simulink model "MSBR_Plant"  (R2021b)
settings: Solver=ode45  StartTime=0.0  StopTime=sim_time  MaxStep=ts_max  RelTol=1e-4
values from neighbouring files (symbols this model uses):
  a_1 = 8.7292e-2/wilson_ratio    (= 0.0087292)    [Whole_Plant_Cool_Pump_Accident_script.m]    (also in Whole_Plant_Fert_Pump_Accident_script.m; Whole_Plant_Fuel_Pump_Accident.m; Whole_Plant_Fuel_Pump_Accident_script.m; Whole_Plant_Reactivity_Accident.m)
  a_2 = 7.3787e-4/wilson_ratio    (= 7.3787e-05)    [Whole_Plant_Cool_Pump_Accident_script.m]    (also in Whole_Plant_Fert_Pump_Accident_script.m; Whole_Plant_Fuel_Pump_Accident.m; Whole_Plant_Fuel_Pump_Accident_script.m; Whole_Plant_Reactivity_Accident.m)
  a_b = 1.656e-5    (= 1.656e-05)    [Whole_Plant_Cool_Pump_Accident_script.m]    (also in Whole_Plant_Fert_Pump_Accident_script.m; Whole_Plant_Fuel_Pump_Accident.m; Whole_Plant_Fuel_Pump_Accident_script.m; Whole_Plant_Reactivity_Accident.m)
  a_f = -8.172e-5    (= -8.172e-05)    [Whole_Plant_Cool_Pump_Accident_script.m]    (also in Whole_Plant_Fert_Pump_Accident_script.m; Whole_Plant_Fuel_Pump_Accident.m; Whole_Plant_Fuel_Pump_Accident_script.m; Whole_Plant_Reactivity_Accident.m)
  a_g = 2.016e-5    (= 2.016e-05)    [Whole_Plant_Cool_Pump_Accident_script.m]    (also in Whole_Plant_Fert_Pump_Accident_script.m; Whole_Plant_Fuel_Pump_Accident.m; Whole_Plant_Fuel_Pump_Accident_script.m; Whole_Plant_Reactivity_Accident.m)
  A_s = pi()*((D_OTSG_i^2)/4) - A_w_OTSG - A_p_OTSG    [Whole_Plant_Cool_Pump_Accident_script.m]    (also in Whole_Plant_Fert_Pump_Accident_script.m; Whole_Plant_Fuel_Pump_Accident.m; Whole_Plant_Fuel_Pump_Accident_script.m; Whole_Plant_Reactivity_Accident.m)
  alpha_co = 316.2    [Whole_Plant_Cool_Pump_Accident_script.m]    (also in Whole_Plant_Fert_Pump_Accident_script.m; Whole_Plant_Fuel_Pump_Accident.m; Whole_Plant_Fuel_Pump_Accident_script.m; Whole_Plant_Reactivity_Accident.m)
  beta = [2.290e-04, 8.320e-04, 7.100e-04, 8.520e-04, 1.710e-04, 1.020e-04]    [Whole_Plant_Cool_Pump_Accident_script.m]    (also in Whole_Plant_Fert_Pump_Accident_script.m; Whole_Plant_Fuel_Pump_Accident.m; Whole_Plant_Fuel_Pump_Accident_script.m; Whole_Plant_Reactivity_Accident.m)
  beta_co = 68.0958    [Whole_Plant_Cool_Pump_Accident_script.m]    (also in Whole_Plant_Fert_Pump_Accident_script.m; Whole_Plant_Fuel_Pump_Accident.m; Whole_Plant_Fuel_Pump_Accident_script.m; Whole_Plant_Reactivity_Accident.m)
  beta_t = sum(beta)    [Whole_Plant_Cool_Pump_Accident_script.m]    (also in Whole_Plant_Fert_Pump_Accident_script.m; Whole_Plant_Fuel_Pump_Accident.m; Whole_Plant_Fuel_Pump_Accident_script.m; Whole_Plant_Reactivity_Accident.m)
  C_nc_X_A_nc = 12.8    [Whole_Plant_Cool_Pump_Accident_script.m]    (also in Whole_Plant_Fert_Pump_Accident_script.m; Whole_Plant_Fuel_Pump_Accident.m; Whole_Plant_Fuel_Pump_Accident_script.m; Whole_Plant_Reactivity_Accident.m)
  C_pcw = 0.0042    [Whole_Plant_Cool_Pump_Accident_script.m]    (also in Whole_Plant_Fert_Pump_Accident_script.m; Whole_Plant_Fuel_Pump_Accident.m; Whole_Plant_Fuel_Pump_Accident_script.m; Whole_Plant_Reactivity_Accident.m)
  C_rh_X_A_rh = 33    [Whole_Plant_Cool_Pump_Accident_script.m]    (also in Whole_Plant_Fert_Pump_Accident_script.m; Whole_Plant_Fuel_Pump_Accident.m; Whole_Plant_Fuel_Pump_Accident_script.m; Whole_Plant_Reactivity_Accident.m)
  C_v = 0.84    [Whole_Plant_Cool_Pump_Accident_script.m]    (also in Whole_Plant_Fert_Pump_Accident_script.m; Whole_Plant_Fuel_Pump_Accident.m; Whole_Plant_Fuel_Pump_Accident_script.m; Whole_Plant_Reactivity_Accident.m)
  ce1 = 1.2471e-07    [Whole_Plant_Cool_Pump_Accident_script.m]    (also in Whole_Plant_Fert_Pump_Accident_script.m; Whole_Plant_Fuel_Pump_Accident.m; Whole_Plant_Fuel_Pump_Accident_script.m; Whole_Plant_Reactivity_Accident.m)
  ce2 = 5.3816e-14    [Whole_Plant_Cool_Pump_Accident_script.m]    (also in Whole_Plant_Fert_Pump_Accident_script.m; Whole_Plant_Fuel_Pump_Accident.m; Whole_Plant_Fuel_Pump_Accident_script.m; Whole_Plant_Reactivity_Accident.m)
  ce3 = 3.3721e-08    [Whole_Plant_Cool_Pump_Accident_script.m]    (also in Whole_Plant_Fert_Pump_Accident_script.m; Whole_Plant_Fuel_Pump_Accident.m; Whole_Plant_Fuel_Pump_Accident_script.m; Whole_Plant_Reactivity_Accident.m)
  Cp_fw = XSteam('Cp_pT',P_set*10,T_fw)/1000    [Whole_Plant_Cool_Pump_Accident_script.m]    (also in Whole_Plant_Fert_Pump_Accident_script.m; Whole_Plant_Fuel_Pump_Accident.m; Whole_Plant_Fuel_Pump_Accident_script.m; Whole_Plant_Reactivity_Accident.m)
  Cp_p = Cp_sec    (= 0.001716588)    [Whole_Plant_Cool_Pump_Accident_script.m]    (also in Whole_Plant_Fert_Pump_Accident_script.m; Whole_Plant_Fuel_Pump_Accident.m; Whole_Plant_Fuel_Pump_Accident_script.m; Whole_Plant_Reactivity_Accident.m)
  Cp_rh = 0.0021520    (= 0.002152)    [Whole_Plant_Cool_Pump_Accident_script.m]    (also in Whole_Plant_Fert_Pump_Accident_script.m; Whole_Plant_Fuel_Pump_Accident.m; Whole_Plant_Fuel_Pump_Accident_script.m; Whole_Plant_Reactivity_Accident.m)
  Cp_s = XSteam('Cp_pT',P_s*10,T_s)/1000    [Whole_Plant_Cool_Pump_Accident_script.m]    (also in Whole_Plant_Fert_Pump_Accident_script.m; Whole_Plant_Fuel_Pump_Accident.m; Whole_Plant_Fuel_Pump_Accident_script.m; Whole_Plant_Reactivity_Accident.m)
  Cp_sc = XSteam('Cp_pT',P_set*10,T_sc2)/1000    [Whole_Plant_Cool_Pump_Accident_script.m]    (also in Whole_Plant_Fert_Pump_Accident_script.m; Whole_Plant_Fuel_Pump_Accident.m; Whole_Plant_Fuel_Pump_Accident_script.m; Whole_Plant_Reactivity_Accident.m)
  Cp_w = 468.992e-6    (= 0.000468992)    [Whole_Plant_Cool_Pump_Accident_script.m]    (also in Whole_Plant_Fert_Pump_Accident_script.m; Whole_Plant_Fuel_Pump_Accident.m; Whole_Plant_Fuel_Pump_Accident_script.m; Whole_Plant_Reactivity_Accident.m)
  D_it = D_ot-2*T_th    (= 0.014147)    [Whole_Plant_Cool_Pump_Accident_script.m]    (also in Whole_Plant_Fert_Pump_Accident_script.m; Whole_Plant_Fuel_Pump_Accident.m; Whole_Plant_Fuel_Pump_Accident_script.m; Whole_Plant_Reactivity_Accident.m)
  D_ot = 0.015875    [Whole_Plant_Cool_Pump_Accident_script.m]    (also in Whole_Plant_Fert_Pump_Accident_script.m; Whole_Plant_Fuel_Pump_Accident.m; Whole_Plant_Fuel_Pump_Accident_script.m; Whole_Plant_Reactivity_Accident.m)
  dHs_dPs = c(1)    [Whole_Plant_Cool_Pump_Accident_script.m]    (also in Whole_Plant_Fert_Pump_Accident_script.m; Whole_Plant_Fuel_Pump_Accident.m; Whole_Plant_Fuel_Pump_Accident_script.m; Whole_Plant_Reactivity_Accident.m)
  eta_hp_isen = 0.861    [Whole_Plant_Cool_Pump_Accident_script.m]    (also in Whole_Plant_Fert_Pump_Accident_script.m; Whole_Plant_Fuel_Pump_Accident.m; Whole_Plant_Fuel_Pump_Accident_script.m; Whole_Plant_Reactivity_Accident.m)
  eta_lp_isen = 0.861    [Whole_Plant_Cool_Pump_Accident_script.m]    (also in Whole_Plant_Fert_Pump_Accident_script.m; Whole_Plant_Fuel_Pump_Accident.m; Whole_Plant_Fuel_Pump_Accident_script.m; Whole_Plant_Reactivity_Accident.m)
  gamma_I = 5.1135e-2    (= 0.051135)    [Whole_Plant_Cool_Pump_Accident_script.m]    (also in Whole_Plant_Fert_Pump_Accident_script.m; Whole_Plant_Fuel_Pump_Accident.m; Whole_Plant_Fuel_Pump_Accident_script.m; Whole_Plant_Reactivity_Accident.m)
  gamma_Xe = 1.1628e-2    (= 0.011628)    [Whole_Plant_Cool_Pump_Accident_script.m]    (also in Whole_Plant_Fert_Pump_Accident_script.m; Whole_Plant_Fuel_Pump_Accident.m; Whole_Plant_Fuel_Pump_Accident_script.m; Whole_Plant_Reactivity_Accident.m)
  H_co0 = 0.149    [Whole_Plant_Cool_Pump_Accident_script.m]    (also in Whole_Plant_Fert_Pump_Accident_script.m; Whole_Plant_Fuel_Pump_Accident.m; Whole_Plant_Fuel_Pump_Accident_script.m; Whole_Plant_Reactivity_Accident.m)
  H_f_co0 = 0.149    [Whole_Plant_Cool_Pump_Accident_script.m]    (also in Whole_Plant_Fert_Pump_Accident_script.m; Whole_Plant_Fuel_Pump_Accident.m; Whole_Plant_Fuel_Pump_Accident_script.m; Whole_Plant_Reactivity_Accident.m)
  H_fg_co0 = 2.35    [Whole_Plant_Cool_Pump_Accident_script.m]    (also in Whole_Plant_Fert_Pump_Accident_script.m; Whole_Plant_Fuel_Pump_Accident.m; Whole_Plant_Fuel_Pump_Accident_script.m; Whole_Plant_Reactivity_Accident.m)
  H_fgrh0 = (XSteam('hV_p', P_s*1e1) - XSteam('hL_p', P_s*1e1))/1e3    [Whole_Plant_Cool_Pump_Accident_script.m]    (also in Whole_Plant_Fert_Pump_Accident_script.m; Whole_Plant_Fuel_Pump_Accident.m; Whole_Plant_Fuel_Pump_Accident_script.m; Whole_Plant_Reactivity_Accident.m)
  H_frh0 = XSteam('hL_p', P_s*1e1)/1e3    [Whole_Plant_Cool_Pump_Accident_script.m]    (also in Whole_Plant_Fert_Pump_Accident_script.m; Whole_Plant_Fuel_Pump_Accident.m; Whole_Plant_Fuel_Pump_Accident_script.m; Whole_Plant_Reactivity_Accident.m)
  h_fwh1 = 0.5927    [Whole_Plant_Cool_Pump_Accident_script.m]    (also in Whole_Plant_Fert_Pump_Accident_script.m; Whole_Plant_Fuel_Pump_Accident.m; Whole_Plant_Fuel_Pump_Accident_script.m; Whole_Plant_Reactivity_Accident.m)
  H_fwh10 = 0.46009    [Whole_Plant_Cool_Pump_Accident_script.m]    (also in Whole_Plant_Fert_Pump_Accident_script.m; Whole_Plant_Fuel_Pump_Accident.m; Whole_Plant_Fuel_Pump_Accident_script.m; Whole_Plant_Reactivity_Accident.m)
  h_fwh2 = 1.230803    [Whole_Plant_Cool_Pump_Accident_script.m]    (also in Whole_Plant_Fert_Pump_Accident_script.m; Whole_Plant_Fuel_Pump_Accident.m; Whole_Plant_Fuel_Pump_Accident_script.m; Whole_Plant_Reactivity_Accident.m)
  H_fwh20 = 0.6784    [Whole_Plant_Cool_Pump_Accident_script.m]    (also in Whole_Plant_Fert_Pump_Accident_script.m; Whole_Plant_Fuel_Pump_Accident.m; Whole_Plant_Fuel_Pump_Accident_script.m; Whole_Plant_Reactivity_Accident.m)
  H_grh0 = 2.8029    [Whole_Plant_Cool_Pump_Accident_script.m]    (also in Whole_Plant_Fert_Pump_Accident_script.m; Whole_Plant_Fuel_Pump_Accident.m; Whole_Plant_Fuel_Pump_Accident_script.m; Whole_Plant_Reactivity_Accident.m)
  H_hp_isen0 = 2.5111    [Whole_Plant_Cool_Pump_Accident_script.m]    (also in Whole_Plant_Fert_Pump_Accident_script.m; Whole_Plant_Fuel_Pump_Accident.m; Whole_Plant_Fuel_Pump_Accident_script.m; Whole_Plant_Reactivity_Accident.m)
  H_hpt_out = 2.6201    [Whole_Plant_Cool_Pump_Accident_script.m]    (also in Whole_Plant_Fert_Pump_Accident_script.m; Whole_Plant_Fuel_Pump_Accident.m; Whole_Plant_Fuel_Pump_Accident_script.m; Whole_Plant_Reactivity_Accident.m)
  H_lp_isen = 958.4*1054.35e-6/0.45359237    (= 2.22774699671)    [Whole_Plant_Cool_Pump_Accident_script.m]    (also in Whole_Plant_Fert_Pump_Accident_script.m; Whole_Plant_Fuel_Pump_Accident.m; Whole_Plant_Fuel_Pump_Accident_script.m; Whole_Plant_Reactivity_Accident.m)
  H_lpt_out = 2.3089    [Whole_Plant_Cool_Pump_Accident_script.m]    (also in Whole_Plant_Fert_Pump_Accident_script.m; Whole_Plant_Fuel_Pump_Accident.m; Whole_Plant_Fuel_Pump_Accident_script.m; Whole_Plant_Reactivity_Accident.m)
  H_nc = XSteam('h_pT', P_s*10, T_s)/1000    [Whole_Plant_Cool_Pump_Accident_script.m]    (also in Whole_Plant_Fert_Pump_Accident_script.m; Whole_Plant_Fuel_Pump_Accident.m; Whole_Plant_Fuel_Pump_Accident_script.m; Whole_Plant_Reactivity_Accident.m)
  h_pw = h_s    (= 0.02555)    [Whole_Plant_Cool_Pump_Accident_script.m]    (also in Whole_Plant_Fert_Pump_Accident_script.m; Whole_Plant_Fuel_Pump_Accident.m; Whole_Plant_Fuel_Pump_Accident_script.m; Whole_Plant_Reactivity_Accident.m)
  H_rh = 2.8115    [Whole_Plant_Cool_Pump_Accident_script.m]    (also in Whole_Plant_Fert_Pump_Accident_script.m; Whole_Plant_Fuel_Pump_Accident.m; Whole_Plant_Fuel_Pump_Accident_script.m; Whole_Plant_Reactivity_Accident.m)
  h_wb = 13349.334646671E-6    (= 0.0133493346467)    [Whole_Plant_Cool_Pump_Accident_script.m]    (also in Whole_Plant_Fert_Pump_Accident_script.m; Whole_Plant_Fuel_Pump_Accident.m; Whole_Plant_Fuel_Pump_Accident_script.m; Whole_Plant_Reactivity_Accident.m)
  h_ws = 5732.378387768E-6    (= 0.00573237838777)    [Whole_Plant_Cool_Pump_Accident_script.m]    (also in Whole_Plant_Fert_Pump_Accident_script.m; Whole_Plant_Fuel_Pump_Accident.m; Whole_Plant_Fuel_Pump_Accident_script.m; Whole_Plant_Reactivity_Accident.m)
  h_wsc = 8385.005556375E-6    (= 0.00838500555638)    [Whole_Plant_Cool_Pump_Accident_script.m]    (also in Whole_Plant_Fert_Pump_Accident_script.m; Whole_Plant_Fuel_Pump_Accident.m; Whole_Plant_Fuel_Pump_Accident_script.m; Whole_Plant_Reactivity_Accident.m)
  hA_bg = A_fert*h_bg    (= 2.76411813627)    [Whole_Plant_Cool_Pump_Accident_script.m]    (also in Whole_Plant_Fert_Pump_Accident_script.m; Whole_Plant_Fuel_Pump_Accident.m; Whole_Plant_Fuel_Pump_Accident_script.m; Whole_Plant_Reactivity_Accident.m)
  hA_co0 = 140    [Whole_Plant_Cool_Pump_Accident_script.m]    (also in Whole_Plant_Fert_Pump_Accident_script.m; Whole_Plant_Fuel_Pump_Accident.m; Whole_Plant_Fuel_Pump_Accident_script.m; Whole_Plant_Reactivity_Accident.m)
  hA_fg_dn = h_fg*A_fuel_down    [Whole_Plant_Cool_Pump_Accident_script.m]    (also in Whole_Plant_Fert_Pump_Accident_script.m; Whole_Plant_Fuel_Pump_Accident.m; Whole_Plant_Fuel_Pump_Accident_script.m; Whole_Plant_Reactivity_Accident.m)
  hA_fg_up = h_fg*A_fuel_up    [Whole_Plant_Cool_Pump_Accident_script.m]    (also in Whole_Plant_Fert_Pump_Accident_script.m; Whole_Plant_Fuel_Pump_Accident.m; Whole_Plant_Fuel_Pump_Accident_script.m; Whole_Plant_Reactivity_Accident.m)
  hA_p_bhx1 = [h_pb*A_pbhx/2,h_pb*A_pbhx/2]    [Whole_Plant_Cool_Pump_Accident_script.m]    (also in Whole_Plant_Fert_Pump_Accident_script.m; Whole_Plant_Fuel_Pump_Accident.m; Whole_Plant_Fuel_Pump_Accident_script.m; Whole_Plant_Reactivity_Accident.m)
  hA_p_bhx2 = hA_p_bhx1    [Whole_Plant_Cool_Pump_Accident_script.m]    (also in Whole_Plant_Fert_Pump_Accident_script.m; Whole_Plant_Fuel_Pump_Accident.m; Whole_Plant_Fuel_Pump_Accident_script.m; Whole_Plant_Reactivity_Accident.m)
  hA_p_bhx3 = hA_p_bhx1    [Whole_Plant_Cool_Pump_Accident_script.m]    (also in Whole_Plant_Fert_Pump_Accident_script.m; Whole_Plant_Fuel_Pump_Accident.m; Whole_Plant_Fuel_Pump_Accident_script.m; Whole_Plant_Reactivity_Accident.m)
  hA_p_bhx4 = hA_p_bhx1    [Whole_Plant_Cool_Pump_Accident_script.m]    (also in Whole_Plant_Fert_Pump_Accident_script.m; Whole_Plant_Fuel_Pump_Accident.m; Whole_Plant_Fuel_Pump_Accident_script.m; Whole_Plant_Reactivity_Accident.m)
  hA_p_fhx1 = [h_p*A_pfhx_dn/2,h_p*A_pfhx_dn/2,h_p*A_pfhx_up/2,h_p*A_pfhx_up/2]    [Whole_Plant_Cool_Pump_Accident_script.m]    (also in Whole_Plant_Fert_Pump_Accident_script.m; Whole_Plant_Fuel_Pump_Accident.m; Whole_Plant_Fuel_Pump_Accident_script.m; Whole_Plant_Reactivity_Accident.m)
  hA_p_fhx2 = hA_p_fhx1    [Whole_Plant_Cool_Pump_Accident_script.m]    (also in Whole_Plant_Fert_Pump_Accident_script.m; Whole_Plant_Fuel_Pump_Accident.m; Whole_Plant_Fuel_Pump_Accident_script.m; Whole_Plant_Reactivity_Accident.m)
  hA_p_fhx3 = hA_p_fhx1    [Whole_Plant_Cool_Pump_Accident_script.m]    (also in Whole_Plant_Fert_Pump_Accident_script.m; Whole_Plant_Fuel_Pump_Accident.m; Whole_Plant_Fuel_Pump_Accident_script.m; Whole_Plant_Reactivity_Accident.m)
  hA_p_fhx4 = hA_p_fhx1    [Whole_Plant_Cool_Pump_Accident_script.m]    (also in Whole_Plant_Fert_Pump_Accident_script.m; Whole_Plant_Fuel_Pump_Accident.m; Whole_Plant_Fuel_Pump_Accident_script.m; Whole_Plant_Reactivity_Accident.m)
  hA_s_bhx1 = [h_sb*A_sbhx/2,h_sb*A_sbhx/2]    [Whole_Plant_Cool_Pump_Accident_script.m]    (also in Whole_Plant_Fert_Pump_Accident_script.m; Whole_Plant_Fuel_Pump_Accident.m; Whole_Plant_Fuel_Pump_Accident_script.m; Whole_Plant_Reactivity_Accident.m)
  hA_s_bhx2 = hA_s_bhx1    [Whole_Plant_Cool_Pump_Accident_script.m]    (also in Whole_Plant_Fert_Pump_Accident_script.m; Whole_Plant_Fuel_Pump_Accident.m; Whole_Plant_Fuel_Pump_Accident_script.m; Whole_Plant_Reactivity_Accident.m)
  hA_s_bhx3 = hA_s_bhx1    [Whole_Plant_Cool_Pump_Accident_script.m]    (also in Whole_Plant_Fert_Pump_Accident_script.m; Whole_Plant_Fuel_Pump_Accident.m; Whole_Plant_Fuel_Pump_Accident_script.m; Whole_Plant_Reactivity_Accident.m)
  hA_s_bhx4 = hA_s_bhx1    [Whole_Plant_Cool_Pump_Accident_script.m]    (also in Whole_Plant_Fert_Pump_Accident_script.m; Whole_Plant_Fuel_Pump_Accident.m; Whole_Plant_Fuel_Pump_Accident_script.m; Whole_Plant_Reactivity_Accident.m)
  hA_s_fhx1 = [h_s*A_sfhx_up/2,h_s*A_sfhx_up/2,h_s*A_sfhx_dn/2,h_s*A_sfhx_dn/2]    [Whole_Plant_Cool_Pump_Accident_script.m]    (also in Whole_Plant_Fert_Pump_Accident_script.m; Whole_Plant_Fuel_Pump_Accident.m; Whole_Plant_Fuel_Pump_Accident_script.m; Whole_Plant_Reactivity_Accident.m)
  hA_s_fhx2 = hA_s_fhx1    [Whole_Plant_Cool_Pump_Accident_script.m]    (also in Whole_Plant_Fert_Pump_Accident_script.m; Whole_Plant_Fuel_Pump_Accident.m; Whole_Plant_Fuel_Pump_Accident_script.m; Whole_Plant_Reactivity_Accident.m)
  hA_s_fhx3 = hA_s_fhx1    [Whole_Plant_Cool_Pump_Accident_script.m]    (also in Whole_Plant_Fert_Pump_Accident_script.m; Whole_Plant_Fuel_Pump_Accident.m; Whole_Plant_Fuel_Pump_Accident_script.m; Whole_Plant_Reactivity_Accident.m)
  hA_s_fhx4 = hA_s_fhx1    [Whole_Plant_Cool_Pump_Accident_script.m]    (also in Whole_Plant_Fert_Pump_Accident_script.m; Whole_Plant_Fuel_Pump_Accident.m; Whole_Plant_Fuel_Pump_Accident_script.m; Whole_Plant_Reactivity_Accident.m)
  I_0 = gamma_I*Sigma_f_msbr*phi_0/lam_I    (= 1.30000734126e+17)    [Whole_Plant_Cool_Pump_Accident_script.m]    (also in Whole_Plant_Fert_Pump_Accident_script.m; Whole_Plant_Fuel_Pump_Accident.m; Whole_Plant_Fuel_Pump_Accident_script.m; Whole_Plant_Reactivity_Accident.m)
  k_1 = 0.5    [Whole_Plant_Cool_Pump_Accident_script.m]    (also in Whole_Plant_Fert_Pump_Accident_script.m; Whole_Plant_Fuel_Pump_Accident.m; Whole_Plant_Fuel_Pump_Accident_script.m; Whole_Plant_Reactivity_Accident.m)
  K_1 = e(1)    [Whole_Plant_Cool_Pump_Accident_script.m]    (also in Whole_Plant_Fert_Pump_Accident_script.m; Whole_Plant_Fuel_Pump_Accident.m; Whole_Plant_Fuel_Pump_Accident_script.m; Whole_Plant_Reactivity_Accident.m)
  k_1b = 0.5    [Whole_Plant_Cool_Pump_Accident_script.m]    (also in Whole_Plant_Fert_Pump_Accident_script.m; Whole_Plant_Fuel_Pump_Accident.m; Whole_Plant_Fuel_Pump_Accident_script.m; Whole_Plant_Reactivity_Accident.m)
  k_2 = 0.5    [Whole_Plant_Cool_Pump_Accident_script.m]    (also in Whole_Plant_Fert_Pump_Accident_script.m; Whole_Plant_Fuel_Pump_Accident.m; Whole_Plant_Fuel_Pump_Accident_script.m; Whole_Plant_Reactivity_Accident.m)
  k_2b = 0.5    [Whole_Plant_Cool_Pump_Accident_script.m]    (also in Whole_Plant_Fert_Pump_Accident_script.m; Whole_Plant_Fuel_Pump_Accident.m; Whole_Plant_Fuel_Pump_Accident_script.m; Whole_Plant_Reactivity_Accident.m)
  k_3 = 0.5    [Whole_Plant_Cool_Pump_Accident_script.m]    (also in Whole_Plant_Fert_Pump_Accident_script.m; Whole_Plant_Fuel_Pump_Accident.m; Whole_Plant_Fuel_Pump_Accident_script.m; Whole_Plant_Reactivity_Accident.m)
  k_4 = 0.5    [Whole_Plant_Cool_Pump_Accident_script.m]    (also in Whole_Plant_Fert_Pump_Accident_script.m; Whole_Plant_Fuel_Pump_Accident.m; Whole_Plant_Fuel_Pump_Accident_script.m; Whole_Plant_Reactivity_Accident.m)
  K_4 = b(1)    [Whole_Plant_Cool_Pump_Accident_script.m]    (also in Whole_Plant_Fert_Pump_Accident_script.m; Whole_Plant_Fuel_Pump_Accident.m; Whole_Plant_Fuel_Pump_Accident_script.m; Whole_Plant_Reactivity_Accident.m)
  K_5 = a(1)    [Whole_Plant_Cool_Pump_Accident_script.m]    (also in Whole_Plant_Fert_Pump_Accident_script.m; Whole_Plant_Fuel_Pump_Accident.m; Whole_Plant_Fuel_Pump_Accident_script.m; Whole_Plant_Reactivity_Accident.m)
  K_b = d(1)    [Whole_Plant_Cool_Pump_Accident_script.m]    (also in Whole_Plant_Fert_Pump_Accident_script.m; Whole_Plant_Fuel_Pump_Accident.m; Whole_Plant_Fuel_Pump_Accident_script.m; Whole_Plant_Reactivity_Accident.m)
  k_b1 = (K_B/2)/K    (= 0.0089463103122)    [Whole_Plant_Cool_Pump_Accident_script.m]    (also in Whole_Plant_Fert_Pump_Accident_script.m; Whole_Plant_Fuel_Pump_Accident.m; Whole_Plant_Fuel_Pump_Accident_script.m; Whole_Plant_Reactivity_Accident.m)
  k_b2 = k_b1    (= 0.0089463103122)    [Whole_Plant_Cool_Pump_Accident_script.m]    (also in Whole_Plant_Fert_Pump_Accident_script.m; Whole_Plant_Fuel_Pump_Accident.m; Whole_Plant_Fuel_Pump_Accident_script.m; Whole_Plant_Reactivity_Accident.m)
  K_bhp = 0.1634    [Whole_Plant_Cool_Pump_Accident_script.m]    (also in Whole_Plant_Fert_Pump_Accident_script.m; Whole_Plant_Fuel_Pump_Accident.m; Whole_Plant_Fuel_Pump_Accident_script.m; Whole_Plant_Reactivity_Accident.m)
  K_blp = 0.2174    [Whole_Plant_Cool_Pump_Accident_script.m]    (also in Whole_Plant_Fert_Pump_Accident_script.m; Whole_Plant_Fuel_Pump_Accident.m; Whole_Plant_Fuel_Pump_Accident_script.m; Whole_Plant_Reactivity_Accident.m)
  k_f1 = ((1 - K_G - K_B - K_Ba)/4)/K    (= 0.226055463576)    [Whole_Plant_Cool_Pump_Accident_script.m]    (also in Whole_Plant_Fert_Pump_Accident_script.m; Whole_Plant_Fuel_Pump_Accident.m; Whole_Plant_Fuel_Pump_Accident_script.m; Whole_Plant_Reactivity_Accident.m)
  k_f2 = k_f1    (= 0.226055463576)    [Whole_Plant_Cool_Pump_Accident_script.m]    (also in Whole_Plant_Fert_Pump_Accident_script.m; Whole_Plant_Fuel_Pump_Accident.m; Whole_Plant_Fuel_Pump_Accident_script.m; Whole_Plant_Reactivity_Accident.m)
  k_f3 = k_f1    (= 0.226055463576)    [Whole_Plant_Cool_Pump_Accident_script.m]    (also in Whole_Plant_Fert_Pump_Accident_script.m; Whole_Plant_Fuel_Pump_Accident.m; Whole_Plant_Fuel_Pump_Accident_script.m; Whole_Plant_Reactivity_Accident.m)
  k_f4 = k_f1    (= 0.226055463576)    [Whole_Plant_Cool_Pump_Accident_script.m]    (also in Whole_Plant_Fert_Pump_Accident_script.m; Whole_Plant_Fuel_Pump_Accident.m; Whole_Plant_Fuel_Pump_Accident_script.m; Whole_Plant_Reactivity_Accident.m)
  k_g1 = ((K_G*K_fuel)/2)/K    (= 0.0346590586566)    [Whole_Plant_Cool_Pump_Accident_script.m]    (also in Whole_Plant_Fert_Pump_Accident_script.m; Whole_Plant_Fuel_Pump_Accident.m; Whole_Plant_Fuel_Pump_Accident_script.m; Whole_Plant_Reactivity_Accident.m)
  k_g2 = k_g1    (= 0.0346590586566)    [Whole_Plant_Cool_Pump_Accident_script.m]    (also in Whole_Plant_Fert_Pump_Accident_script.m; Whole_Plant_Fuel_Pump_Accident.m; Whole_Plant_Fuel_Pump_Accident_script.m; Whole_Plant_Reactivity_Accident.m)
  k_g3 = (K_G*(1-K_fuel))/K    (= 0.00856740775781)    [Whole_Plant_Cool_Pump_Accident_script.m]    (also in Whole_Plant_Fert_Pump_Accident_script.m; Whole_Plant_Fuel_Pump_Accident.m; Whole_Plant_Fuel_Pump_Accident_script.m; Whole_Plant_Reactivity_Accident.m)
  K_sc = f(1)    [Whole_Plant_Cool_Pump_Accident_script.m]    (also in Whole_Plant_Fert_Pump_Accident_script.m; Whole_Plant_Fuel_Pump_Accident.m; Whole_Plant_Fuel_Pump_Accident_script.m; Whole_Plant_Reactivity_Accident.m)
  L = 22.0    (= 22)    [Whole_Plant_Cool_Pump_Accident_script.m]    (also in Whole_Plant_Fert_Pump_Accident_script.m; Whole_Plant_Fuel_Pump_Accident.m; Whole_Plant_Fuel_Pump_Accident_script.m; Whole_Plant_Reactivity_Accident.m)
  L_b = 1.9    [Whole_Plant_Cool_Pump_Accident_script.m]    (also in Whole_Plant_Fert_Pump_Accident_script.m; Whole_Plant_Fuel_Pump_Accident.m; Whole_Plant_Fuel_Pump_Accident_script.m; Whole_Plant_Reactivity_Accident.m)
  L_s = 16.53    [Whole_Plant_Cool_Pump_Accident_script.m]    (also in Whole_Plant_Fert_Pump_Accident_script.m; Whole_Plant_Fuel_Pump_Accident.m; Whole_Plant_Fuel_Pump_Accident_script.m; Whole_Plant_Reactivity_Accident.m)
  L_sc = L-L_b-L_s    (= 3.57)    [Whole_Plant_Cool_Pump_Accident_script.m]    (also in Whole_Plant_Fert_Pump_Accident_script.m; Whole_Plant_Fuel_Pump_Accident.m; Whole_Plant_Fuel_Pump_Accident_script.m; Whole_Plant_Reactivity_Accident.m)
  Lam = 3.3e-4    (= 0.00033)    [Whole_Plant_Cool_Pump_Accident_script.m]    (also in Whole_Plant_Fert_Pump_Accident_script.m; Whole_Plant_Fuel_Pump_Accident.m; Whole_Plant_Fuel_Pump_Accident_script.m; Whole_Plant_Reactivity_Accident.m)
  lam = [1.260e-02, 3.370e-02, 1.390e-01, 3.250e-01, 1.130e+00, 2.500e+00]    [Whole_Plant_Cool_Pump_Accident_script.m]    (also in Whole_Plant_Fert_Pump_Accident_script.m; Whole_Plant_Fuel_Pump_Accident.m; Whole_Plant_Fuel_Pump_Accident_script.m; Whole_Plant_Reactivity_Accident.m)
  lam_bubl = 2.0e-2    (= 0.02)    [Whole_Plant_Cool_Pump_Accident_script.m]    (also in Whole_Plant_Fert_Pump_Accident_script.m; Whole_Plant_Fuel_Pump_Accident.m; Whole_Plant_Fuel_Pump_Accident_script.m; Whole_Plant_Reactivity_Accident.m)
  lam_I = 2.875e-5    (= 2.875e-05)    [Whole_Plant_Cool_Pump_Accident_script.m]    (also in Whole_Plant_Fert_Pump_Accident_script.m; Whole_Plant_Fuel_Pump_Accident.m; Whole_Plant_Fuel_Pump_Accident_script.m; Whole_Plant_Reactivity_Accident.m)
  lam_Xe = 2.0916e-5    (= 2.0916e-05)    [Whole_Plant_Cool_Pump_Accident_script.m]    (also in Whole_Plant_Fert_Pump_Accident_script.m; Whole_Plant_Fuel_Pump_Accident.m; Whole_Plant_Fuel_Pump_Accident_script.m; Whole_Plant_Reactivity_Accident.m)
  m_bm = (W_b1+W_b2+W_b3+W_b4)*time_mixb    (= 2167.1636)    [Whole_Plant_Cool_Pump_Accident_script.m]    (also in Whole_Plant_Fert_Pump_Accident_script.m; Whole_Plant_Fuel_Pump_Accident.m; Whole_Plant_Fuel_Pump_Accident_script.m; Whole_Plant_Reactivity_Accident.m)
  M_cw = 65000    [Whole_Plant_Cool_Pump_Accident_script.m]    (also in Whole_Plant_Fert_Pump_Accident_script.m; Whole_Plant_Fuel_Pump_Accident.m; Whole_Plant_Fuel_Pump_Accident_script.m; Whole_Plant_Reactivity_Accident.m)
  m_fm = (W_f1+W_f2+W_f3+W_f4)*time_mixf    (= 5443.108)    [Whole_Plant_Cool_Pump_Accident_script.m]    (also in Whole_Plant_Fert_Pump_Accident_script.m; Whole_Plant_Fuel_Pump_Accident.m; Whole_Plant_Fuel_Pump_Accident_script.m; Whole_Plant_Reactivity_Accident.m)
  M_hw0 = 10000    [Whole_Plant_Cool_Pump_Accident_script.m]    (also in Whole_Plant_Fert_Pump_Accident_script.m; Whole_Plant_Fuel_Pump_Accident.m; Whole_Plant_Fuel_Pump_Accident_script.m; Whole_Plant_Reactivity_Accident.m)
  m_sm = (W_s1+W_s2+W_s3+W_s4)*time_mixs    (= 8467.056)    [Whole_Plant_Cool_Pump_Accident_script.m]    (also in Whole_Plant_Fert_Pump_Accident_script.m; Whole_Plant_Fuel_Pump_Accident.m; Whole_Plant_Fuel_Pump_Accident_script.m; Whole_Plant_Reactivity_Accident.m)
  M_stm = 0.018    [Whole_Plant_Cool_Pump_Accident_script.m]    (also in Whole_Plant_Fert_Pump_Accident_script.m; Whole_Plant_Fuel_Pump_Accident.m; Whole_Plant_Fuel_Pump_Accident_script.m; Whole_Plant_Reactivity_Accident.m)
  mcp_b1 = mass_bn*Cp_b    (= 4.17494922705)    [Whole_Plant_Cool_Pump_Accident_script.m]    (also in Whole_Plant_Fert_Pump_Accident_script.m; Whole_Plant_Fuel_Pump_Accident.m; Whole_Plant_Fuel_Pump_Accident_script.m; Whole_Plant_Reactivity_Accident.m)
  mcp_b2 = mcp_b1    (= 4.17494922705)    [Whole_Plant_Cool_Pump_Accident_script.m]    (also in Whole_Plant_Fert_Pump_Accident_script.m; Whole_Plant_Fuel_Pump_Accident.m; Whole_Plant_Fuel_Pump_Accident_script.m; Whole_Plant_Reactivity_Accident.m)
  mcp_f1 = mass_fn*Cp_f    (= 5.5019469141)    [Whole_Plant_Cool_Pump_Accident_script.m]    (also in Whole_Plant_Fert_Pump_Accident_script.m; Whole_Plant_Fuel_Pump_Accident.m; Whole_Plant_Fuel_Pump_Accident_script.m; Whole_Plant_Reactivity_Accident.m)
  mcp_f2 = mass_fn*Cp_f    (= 5.5019469141)    [Whole_Plant_Cool_Pump_Accident_script.m]    (also in Whole_Plant_Fert_Pump_Accident_script.m; Whole_Plant_Fuel_Pump_Accident.m; Whole_Plant_Fuel_Pump_Accident_script.m; Whole_Plant_Reactivity_Accident.m)
  mcp_f3 = mass_fn*Cp_f    (= 5.5019469141)    [Whole_Plant_Cool_Pump_Accident_script.m]    (also in Whole_Plant_Fert_Pump_Accident_script.m; Whole_Plant_Fuel_Pump_Accident.m; Whole_Plant_Fuel_Pump_Accident_script.m; Whole_Plant_Reactivity_Accident.m)
  mcp_f4 = mass_fn*Cp_f    (= 5.5019469141)    [Whole_Plant_Cool_Pump_Accident_script.m]    (also in Whole_Plant_Fert_Pump_Accident_script.m; Whole_Plant_Fuel_Pump_Accident.m; Whole_Plant_Fuel_Pump_Accident_script.m; Whole_Plant_Reactivity_Accident.m)
  mcp_g1 = (mass_grap*Cp_g)*K_fuel/2    (= 32.9814988203)    [Whole_Plant_Cool_Pump_Accident_script.m]    (also in Whole_Plant_Fert_Pump_Accident_script.m; Whole_Plant_Fuel_Pump_Accident.m; Whole_Plant_Fuel_Pump_Accident_script.m; Whole_Plant_Reactivity_Accident.m)
  mcp_g2 = mcp_g1    (= 32.9814988203)    [Whole_Plant_Cool_Pump_Accident_script.m]    (also in Whole_Plant_Fert_Pump_Accident_script.m; Whole_Plant_Fuel_Pump_Accident.m; Whole_Plant_Fuel_Pump_Accident_script.m; Whole_Plant_Reactivity_Accident.m)
  mcp_g3 = (mass_grap*Cp_g)*(1-K_fuel)    (= 8.15273004546)    [Whole_Plant_Cool_Pump_Accident_script.m]    (also in Whole_Plant_Fert_Pump_Accident_script.m; Whole_Plant_Fuel_Pump_Accident.m; Whole_Plant_Fuel_Pump_Accident_script.m; Whole_Plant_Reactivity_Accident.m)
  mcp_p_bhx1 = mp_bhx1*Cp_b    [Whole_Plant_Cool_Pump_Accident_script.m]    (also in Whole_Plant_Fert_Pump_Accident_script.m; Whole_Plant_Fuel_Pump_Accident.m; Whole_Plant_Fuel_Pump_Accident_script.m; Whole_Plant_Reactivity_Accident.m)
  mcp_p_bhx2 = mp_bhx2*Cp_b    [Whole_Plant_Cool_Pump_Accident_script.m]    (also in Whole_Plant_Fert_Pump_Accident_script.m; Whole_Plant_Fuel_Pump_Accident.m; Whole_Plant_Fuel_Pump_Accident_script.m; Whole_Plant_Reactivity_Accident.m)
  mcp_p_bhx3 = mp_bhx3*Cp_b    [Whole_Plant_Cool_Pump_Accident_script.m]    (also in Whole_Plant_Fert_Pump_Accident_script.m; Whole_Plant_Fuel_Pump_Accident.m; Whole_Plant_Fuel_Pump_Accident_script.m; Whole_Plant_Reactivity_Accident.m)
  ... (+213 more)
undefined symbols (not defined in the file or in its folder): C0, H_con_table, H_convap_table, H_rh_table, H_rh_table1, H_rh_table2, H_rhvap_table, H_s_table, H_table, P_con_table, P_nc_table, P_rh_table, P_rh_table1, pres_table, rho_rh_table, rho_table, SV_nc_table, SVf_nc_table, temp_table
(part 2 of 13)

== system MSBR_Plant/Balance of Plant (BOP)/HIGH PRESSURE TURBINE ==
  Steam Flow Rate Nozzle Chest : Inport
  Steam Enthalpy Nozzle Chest : Inport  Port=2
  Steam Pressure Nozzle Chest : Inport  Port=3
  Steam Pressure Reheater : Inport  Port=4
  Constant : Constant  Value=tau_hpt
  Constant1 : Constant  Value=K_bhp
  Constant2 : Constant  Value=eta_hp_isen
  Constant3 : Constant  Value=term1
  Constant4 : Constant  Value=ce1
  Constant5 : Constant  Value=ce2
  Constant6 : Constant  Value=p1
  Constant7 : Constant  Value=p2
  Constant8 : Constant  Value=ce3
  Divide : Product  Inputs=*/
  Divide1 : Product  Inputs=**
  Divide2 : Product  Inputs=**
  Minus : Sum  Inputs=+--
  Minus1 : Sum  Inputs=+-
  Minus2 : Sum
  Minus3 : Sum  Inputs=++--
  Minus4 : Sum  Inputs=+-
  Minus5 : Sum  Inputs=+-
  Mux1 : Mux  Inputs=8
  Product : Product
  Product1 : Product
  Product2 : Product
  Square : Math  Operator=square  SaturateOnIntegerOverflow=on
  To Workspace1 : ToWorkspace  VariableName=HPT_mux  SaveFormat=Timeseries  SampleTime=-1
      settings: Save2DSignal=2-D array (concatenate along first dimension)
  Unit Delay1 : UnitDelay  InitialCondition=H_hpt_out  SampleTime=-1  HasFrameUpgradeWarning=on
  Unit Delay2 : UnitDelay  InitialCondition=H_hp_isen0  SampleTime=-1  HasFrameUpgradeWarning=on
  Unit Delay3 : UnitDelay  InitialCondition=w_bhp_out  SampleTime=-1  HasFrameUpgradeWarning=on
  W_hpt : Integrator  InitialCondition=w_hp_out
  Steam Flow Rate HP Turbine : Outport  VectorParamsAs1DForOutWhenUnconnected=off
  Steam Bleed Flow HP Turbine : Outport  Port=2  VectorParamsAs1DForOutWhenUnconnected=off
  Steam Enthalpy HP Turbine : Outport  Port=3  VectorParamsAs1DForOutWhenUnconnected=off
  wires:
  Steam Flow Rate Nozzle Chest/1 -> [W_nc]
  Steam Enthalpy Nozzle Chest/1 -> [H_nc]
  Steam Pressure Nozzle Chest/1 -> [P_nc]
  Steam Pressure Reheater/1 -> [P_rh]
  W_hpt/1 -> [W_hpt]
  Unit Delay3/1 -> [W_bhp]
  Unit Delay1/1 -> [H_hpt]
  Unit Delay2/1 -> [H_hp_isen]
  [W_hpt] -> Steam Flow Rate HP Turbine/1
  [W_bhp] -> Steam Bleed Flow HP Turbine/1
  [H_hpt] -> Steam Enthalpy HP Turbine/1
  Mux1/1 -> To Workspace1/1
  [W_nc] -> Minus/1
  [W_bhp] -> Minus/2
  [W_hpt] -> Minus/3
  Minus/1 -> Divide/1
  Divide/1 -> W_hpt/1
  [tau_hpt] -> Divide/2
  Constant/1 -> [tau_hpt]
  Constant1/1 -> [K_bhp]
  [K_bhp] -> Divide1/1
  Divide1/1 -> Unit Delay3/1
  [W_nc] -> Divide1/2
  Constant2/1 -> [eta_hp_isen]
  [H_nc] -> Minus1/2
  [H_hp_isen] -> Minus1/1
  Minus1/1 -> Divide2/1
  [eta_hp_isen] -> Divide2/2
  Divide2/1 -> Minus2/2
  Minus2/1 -> Unit Delay1/1
  [H_nc] -> Minus2/1
  Constant4/1 -> [ce1]
  Constant5/1 -> [ce2]
  Constant3/1 -> [term1]
  Constant7/1 -> [p2]
  Constant6/1 -> [p1]
  Constant8/1 -> [ce3]
  Minus3/1 -> Unit Delay2/1
  [term1] -> Minus3/1
  Product/1 -> Minus3/2
  [ce1] -> Product/1
  Minus4/1 -> Square/1, Product/2
  [P_rh] -> Minus4/1
  [p1] -> Minus4/2
  Square/1 -> Product1/1
  [ce2] -> Product1/2
  Product1/1 -> Minus3/3
  [P_nc] -> Minus5/1
  [p2] -> Minus5/2
  Minus5/1 -> Product2/2
  [ce3] -> Product2/1
  Product2/1 -> Minus3/4
  [W_nc] -> Mux1/1
  [H_nc] -> Mux1/2
  [P_nc] -> Mux1/3
  [P_rh] -> Mux1/4
  [W_hpt] -> Mux1/5
  [W_bhp] -> Mux1/6
  [H_hpt] -> Mux1/7
  [H_hp_isen] -> Mux1/8

== system MSBR_Plant/Balance of Plant (BOP)/LOW PRESSURE TURBINE ==
  Flow from Reheater : Inport
  Steam Enthalpy Reheater : Inport  Port=2
  Constant : Constant  Value=tau_lpt
  Constant1 : Constant  Value=K_blp
  Constant2 : Constant  Value=eta_lp_isen
  Constant3 : Constant  Value=H_lp_isen
  Divide : Product  Inputs=*/
  Divide1 : Product  Inputs=**
  Divide2 : Product  Inputs=**
  Minus : Sum  Inputs=+--
  Minus1 : Sum  Inputs=+-
  Minus2 : Sum  Inputs=+-
  Mux1 : Mux  Inputs=5
  Scope : Scope
  Scope1 : Scope
  To Workspace1 : ToWorkspace  VariableName=LPT_mux  SaveFormat=Timeseries  SampleTime=-1
      settings: Save2DSignal=2-D array (concatenate along first dimension)
  Unit Delay1 : UnitDelay  InitialCondition=H_lpt_out  SampleTime=-1  HasFrameUpgradeWarning=on
  Unit Delay3 : UnitDelay  InitialCondition=123.6368  SampleTime=-1  HasFrameUpgradeWarning=on
  W_lpt : Integrator  InitialCondition=w_lp_out
  Steam Flow Rate LP Turbine : Outport  VectorParamsAs1DForOutWhenUnconnected=off
  Steam Bleed Flow Rate LP Turbine : Outport  Port=2  VectorParamsAs1DForOutWhenUnconnected=off
  Steam Enthalpy LP Turbine : Outport  Port=3  VectorParamsAs1DForOutWhenUnconnected=off
  wires:
  Flow from Reheater/1 -> [W_rh]
  Steam Enthalpy Reheater/1 -> [H_rh]
  W_lpt/1 -> Scope/1, [W_lpt]
  Unit Delay3/1 -> [W_blp]
  Unit Delay1/1 -> [H_lpt]
  [W_lpt] -> Steam Flow Rate LP Turbine/1
  [W_blp] -> Steam Bleed Flow Rate LP Turbine/1
  [H_lpt] -> Steam Enthalpy LP Turbine/1
  [W_lpt] -> Mux1/3
  Mux1/1 -> To Workspace1/1
  Constant/1 -> [tau_lpt]
  Constant1/1 -> [K_blp]
  Constant2/1 -> [eta_lp_isen]
  Constant3/1 -> [H_lp_isen]
  Minus/1 -> Divide/1
  Divide/1 -> Scope1/1, W_lpt/1
  [W_rh] -> Minus/1
  [W_lpt] -> Minus/3
  [W_blp] -> Minus/2
  [tau_lpt] -> Divide/2
  [K_blp] -> Divide1/1
  [W_rh] -> Divide1/2
  Divide1/1 -> Unit Delay3/1
  [H_rh] -> Minus1/1
  Minus2/1 -> Divide2/2
  [eta_lp_isen] -> Divide2/1
  [H_rh] -> Minus2/1
  [H_lp_isen] -> Minus2/2
  Divide2/1 -> Minus1/2
  Minus1/1 -> Unit Delay1/1
  [W_rh] -> Mux1/1
  [H_rh] -> Mux1/2
  [W_blp] -> Mux1/4
  [H_lpt] -> Mux1/5

== system MSBR_Plant/Balance of Plant (BOP)/MOISTURE SEPARATOR ==
  Enthalpy of Vaporization : Inport
  Enthalpy of Reheater Feedwater : Inport  Port=2
  Steam Flow Rate Nozzle Chest : Inport  Port=3
  Steam Flow Rate HP Turbine : Inport  Port=4
  Steam Bleed Flow HP Turbine : Inport  Port=5
  Steam Enthalpy HP Turbine : Inport  Port=6
  Divide : Product  Inputs=*/
  Minus : Sum  Inputs=+--
  Minus1 : Sum  Inputs=+-
  Mux1 : Mux  Inputs=8
  Product : Product
  To Workspace : ToWorkspace  VariableName=MS_mux  SaveFormat=Timeseries  SampleTime=-1
      settings: Save2DSignal=2-D array (concatenate along first dimension)
  Flow to Heater 2 : Outport  VectorParamsAs1DForOutWhenUnconnected=off
  Flow to Reheater : Outport  Port=2  VectorParamsAs1DForOutWhenUnconnected=off
  wires:
  Enthalpy of Vaporization/1 -> [H_fg]
  Enthalpy of Reheater Feedwater/1 -> [H_f]
  Steam Flow Rate Nozzle Chest/1 -> [W_nc]
  Steam Flow Rate HP Turbine/1 -> [W_hpt]
  Steam Bleed Flow HP Turbine/1 -> [W_bhp]
  Steam Enthalpy HP Turbine/1 -> [H_hpt]
  [W_liq] -> Flow to Heater 2/1
  [W_ms] -> Flow to Reheater/1
  Mux1/1 -> To Workspace/1
  [H_fg] -> Mux1/1
  [H_f] -> Mux1/2
  [W_nc] -> Mux1/3
  [W_hpt] -> Mux1/4
  [W_bhp] -> Mux1/5
  [H_hpt] -> Mux1/6
  [W_liq] -> Mux1/7
  [W_ms] -> Mux1/8
  [W_nc] -> Minus/1
  [W_bhp] -> Minus/2
  [W_ms] -> Minus/3
  Minus/1 -> [W_liq]
  Minus1/1 -> Divide/1
  Divide/1 -> Product/1
  [H_hpt] -> Minus1/1
  [H_f] -> Minus1/2
  [H_fg] -> Divide/2
  [W_hpt] -> Product/2
  Product/1 -> [W_ms]

== system MSBR_Plant/Balance of Plant (BOP)/NOZZLE CHEST ==
  note: Represents the product of C_nc (flow coefficient of nozzle chest) and A_nc (area of nozzle chest)
  Steam Flow Rate OTSG : Inport
  Steam Enthalpy OTSG : Inport  Port=2
  Steam Enthalpy HP Turbine : Inport  Port=3
  Steam Pressure Reheater : Inport  Port=4
  Constant : Constant  Value=V_nc
  Constant3 : Constant
  Constant4 : Constant
  Constant5 : Constant  Value=C_nc_X_A_nc
  Divide{,2,6..7} (4 alike) : Product  Inputs=*/
  Divide1 : Product  Inputs=**/
  Divide{3..5,8} (4 alike) : Product  Inputs=**
  Flow Rate out of Nozzle Chest : Scope
  Fluid enthalpy and Enthalpy of Vaporization for Reheater : Scope  NumInputPorts=2
  H_nc : Integrator  InitialCondition=H_nc
  Minus{,1..3,5} (5 alike) : Sum  Inputs=+-
  Minus4 : Sum
  Mux1 : Mux  Inputs=15
  NC Pressure : Lookup_n-D  BreakpointsForDimension1=H_table  BreakpointsForDimension2=rho_table  Table=P_nc_table  InternalRulePriority=Speed  RndMeth=Simplest  InputSameDT=on
      settings: InputPortMap=u0,u1
  Nozzle chest and HPT Density : Scope  NumInputPorts=2
  Nozzle chest and Reheater Pressure : Scope  NumInputPorts=2
  Plus : Sum
  Product{,1..3} (4 alike) : Product
  RH Fluid Specific Volume : Lookup_n-D  NumberOfTableDimensions=1  BreakpointsForDimension1=P_rh_table1  Table=SVf_nc_table  InternalRulePriority=Speed  RndMeth=Simplest  InputSameDT=on
  RH H_liq : Lookup_n-D  NumberOfTableDimensions=1  BreakpointsForDimension1=P_rh_table1  Table=H_rh_table  InternalRulePriority=Speed  RndMeth=Simplest  InputSameDT=on
  RH H_vaporization : Lookup_n-D  NumberOfTableDimensions=1  BreakpointsForDimension1=P_rh_table1  Table=H_rhvap_table  InternalRulePriority=Speed  RndMeth=Simplest  InputSameDT=on
  RH Vapor Specific Volume : Lookup_n-D  NumberOfTableDimensions=1  BreakpointsForDimension1=P_rh_table1  Table=SV_nc_table  InternalRulePriority=Speed  RndMeth=Simplest  InputSameDT=on
  Scope{,1..7} (8 alike) : Scope
  Sqrt : Sqrt  SaturateOnIntegerOverflow=on
  Square : Math  Operator=square  SaturateOnIntegerOverflow=on
  To Workspace1 : ToWorkspace  VariableName=NC_mux  SaveFormat=Timeseries  SampleTime=-1
      settings: Save2DSignal=2-D array (concatenate along first dimension)
  Unit Delay1 : UnitDelay  InitialCondition=H_fgrh0  SampleTime=-1  HasFrameUpgradeWarning=on
  Unit Delay2 : UnitDelay  InitialCondition=H_frh0  SampleTime=-1  HasFrameUpgradeWarning=on
  Unit Delay3 : UnitDelay  InitialCondition=nu_g0  SampleTime=-1  HasFrameUpgradeWarning=on
  Unit Delay4 : UnitDelay  SampleTime=-1  HasFrameUpgradeWarning=on
  Unit Delay5 : UnitDelay  InitialCondition=266.6348  SampleTime=-1  HasFrameUpgradeWarning=on
  Unit Delay6 : UnitDelay  InitialCondition=nu_f0  SampleTime=-1  HasFrameUpgradeWarning=on
  rho_nc : Integrator  InitialCondition=rho_nc  UpperSaturationLimit=rho_nc
  Enthalpy of Vaporization : Outport  VectorParamsAs1DForOutWhenUnconnected=off
  Enthalpy of Reheater Feedwater : Outport  Port=2  VectorParamsAs1DForOutWhenUnconnected=off
  Steam Flow Rate in Nozzle Chest : Outport  Port=3  VectorParamsAs1DForOutWhenUnconnected=off
  Steam Enthalpy in Nozzle Chest : Outport  Port=4  VectorParamsAs1DForOutWhenUnconnected=off
  Steam Pressure in Nozzle Chest : Outport  Port=5  VectorParamsAs1DForOutWhenUnconnected=off
  wires:
  Steam Flow Rate OTSG/1 -> [W_in]
  Steam Enthalpy OTSG/1 -> [H_in]
  Steam Enthalpy HP Turbine/1 -> [H_hpt]
  Steam Pressure Reheater/1 -> [P_rh]
  NC Pressure/1 -> [P_nc]
  RH Vapor Specific Volume/1 -> Unit Delay3/1
  RH H_liq/1 -> Unit Delay2/1
  RH H_vaporization/1 -> Unit Delay1/1
  Unit Delay1/1 -> [H_fg_P_rh]
  rho_nc/1 -> [rho_nc]
  Unit Delay2/1 -> [H_f_P_rh]
  Unit Delay3/1 -> [nu_g]
  Unit Delay4/1 -> [drho_nc_dt]
  [W_nc] -> Steam Flow Rate in Nozzle Chest/1
  [H_f_P_rh] -> Enthalpy of Reheater Feedwater/1
  [H_fg_P_rh] -> Enthalpy of Vaporization/1
  [H_nc] -> Steam Enthalpy in Nozzle Chest/1
  [P_nc] -> Steam Pressure in Nozzle Chest/1
  [W_in] -> Mux1/1
  [H_in] -> Mux1/2
  [H_hpt] -> Mux1/3
  [P_rh] -> Nozzle chest and Reheater Pressure/2, Mux1/4
  [H_nc] -> Mux1/6
  [dH_nc_dt] -> Mux1/5
  [drho_nc_dt] -> Mux1/7
  [rho_nc] -> Nozzle chest and HPT Density/1, Mux1/8
  Mux1/1 -> Unit Delay5/1
  Unit Delay5/1 -> To Workspace1/1
  [W_nc] -> Flow Rate out of Nozzle Chest/1, Mux1/9
  [P_nc] -> Mux1/10, Nozzle chest and Reheater Pressure/1
  [X] -> Mux1/11
  [nu_g] -> Mux1/13
  [H_f_P_rh] -> Fluid enthalpy and Enthalpy of Vaporization for Reheater/1, Mux1/14
  [H_fg_P_rh] -> Fluid enthalpy and Enthalpy of Vaporization for Reheater/2, Mux1/15
  Constant/1 -> [V_nc]
  Product/1 -> Minus/1
  [W_in] -> Product/1
  [H_in] -> Product/2
  Product1/1 -> Minus/2
  [W_nc] -> Product1/1
  [H_nc] -> Product1/2
  [V_nc] -> Product2/2
  Minus/1 -> Divide/1
  [rho_nc] -> Product2/1
  Product2/1 -> Divide/2
  Divide/1 -> Plus/1
  [rho_nc] -> Square/1
  Divide1/1 -> Plus/2
  [P_nc] -> Divide1/1
  [drho_nc_dt] -> Divide1/2
  Square/1 -> Divide1/3
  Plus/1 -> H_nc/1, [dH_nc_dt]
  H_nc/1 -> [H_nc]
  Divide2/1 -> rho_nc/1, Unit Delay4/1
  [W_in] -> Scope6/1, Minus1/1
  [W_nc] -> Scope7/1, Minus1/2
  [V_nc] -> Divide2/2
  Minus1/1 -> Divide2/1
  [C_nc_X_A_nc] -> Divide3/1
  Sqrt/1 -> Divide3/2
  Minus2/1 -> Sqrt/1
  Divide4/1 -> Scope/1, Minus2/1
  Divide5/1 -> Scope1/1, Minus2/2
  [P_nc] -> Scope2/1, Divide4/1
  [rho_nc] -> Scope5/1, Divide4/2
  [rho_hpt] -> Scope4/1, Divide5/2
  [P_rh] -> Scope3/1, Divide5/1
  [rho_hpt] -> Nozzle chest and HPT Density/2, Mux1/12
  Divide3/1 -> [W_nc]
  [H_nc] -> NC Pressure/1
  [rho_nc] -> NC Pressure/2
  [H_hpt] -> Minus3/1
  [H_f_P_rh] -> Minus3/2
  Minus3/1 -> Divide6/1
  [H_fg_P_rh] -> Divide6/2
  Divide6/1 -> [X]
  Constant3/1 -> Divide7/1
  Divide7/1 -> [rho_hpt]
  [X] -> Product3/1
  [nu_g] -> Product3/2
  Product3/1 -> Minus4/1
  Minus4/1 -> Divide7/2
  Constant4/1 -> Minus5/1
  [X] -> Minus5/2
  Minus5/1 -> Divide8/1
  [nu_f] -> Divide8/2
  Divide8/1 -> Minus4/2
  [P_rh] -> RH Vapor Specific Volume/1
  [P_rh] -> RH H_liq/1
  [P_rh] -> RH H_vaporization/1
  Constant5/1 -> [C_nc_X_A_nc]
  [P_rh] -> RH Fluid Specific Volume/1
  Unit Delay6/1 -> [nu_f]
  RH Fluid Specific Volume/1 -> Unit Delay6/1

== system MSBR_Plant/Balance of Plant (BOP)/REHEATER ==
  note: Constant is the product of C_rh and A_rh (Coefficient of flow in rh and Area of rh)
  Steam Flow Rate Secondary Valve : Inport
  Flow from Moisture Seperator Reheater : Inport  Port=2
  Steam Temperature : Inport  Port=3
  Constant : Constant  Value=V_rh
  Constant1 : Constant  Value=C_rh_X_A_rh
  Constant2 : Constant  Value=tau_rht
  Constant3 : Constant  Value=Cp_rh
  Constant4 : Constant  Value=2
  Constant5 : Constant  Value=tau_rhs
  Constant6 : Constant  Value=M_stm
  Constant7 : Constant  Value=R
  Constant8 : Constant  Value=0.75
  Divide{,1,3,5,7} (5 alike) : Product  Inputs=*/
  Divide2 : Product  Inputs=**/
  Divide4 : Product  Inputs=***//
  Divide6 : Product  Inputs=***
  H_rh : Integrator  InitialCondition=H_rh
  Minus{,2,4,6..7} (5 alike) : Sum  Inputs=+-
  Minus1 : Sum
  Minus3 : Sum  Inputs=++-
  Minus5 : Sum
  Mux1 : Mux  Inputs=12
  Product{,1..6} (7 alike) : Product
  Q_rh : Integrator  InitialCondition=Q_rh
  RH H_liq : Lookup_n-D  NumberOfTableDimensions=1  BreakpointsForDimension1=P_rh_table1  Table=H_rh_table1  InternalRulePriority=Speed  RndMeth=Simplest  InputSameDT=on
  RH Pressure : Lookup_n-D  BreakpointsForDimension1=H_rh_table2  BreakpointsForDimension2=rho_rh_table  Table=P_rh_table  InternalRulePriority=Speed  RndMeth=Simplest  InputSameDT=on
      settings: InputPortMap=u0,u1
  Sqrt : Sqrt  SaturateOnIntegerOverflow=on
  Square : Math  Operator=square  SaturateOnIntegerOverflow=on
  To Workspace : ToWorkspace  VariableName=RH_mux  SaveFormat=Timeseries  SampleTime=-1
      settings: Save2DSignal=2-D array (concatenate along first dimension)
  Unit Delay1 : UnitDelay  InitialCondition=w_rh_out  SampleTime=-1  HasFrameUpgradeWarning=on
  Unit Delay2 : UnitDelay  InitialCondition=H_grh0  SampleTime=-1  HasFrameUpgradeWarning=on
  Unit Delay3 : UnitDelay  InitialCondition=T_rh0  SampleTime=-1  HasFrameUpgradeWarning=on
  Unit Delay7 : UnitDelay  InitialCondition=P_rh0  SampleTime=-1  HasFrameUpgradeWarning=on
  W_vrh : Integrator  InitialCondition=w_vrh_out
  rho_rh : Integrator  InitialCondition=rho_rh
  Flow to LP Turbine : Outport  VectorParamsAs1DForOutWhenUnconnected=off
  Flow to Feedwater Heater 2 : Outport  Port=2  VectorParamsAs1DForOutWhenUnconnected=off
  Steam Pressure Reheater : Outport  Port=3  VectorParamsAs1DForOutWhenUnconnected=off
  Steam Enthalpy Reheater : Outport  Port=4  VectorParamsAs1DForOutWhenUnconnected=off
  wires:
  Steam Flow Rate Secondary Valve/1 -> [W_v]
  Flow from Moisture Seperator Reheater/1 -> [W_ms]
  Steam Temperature/1 -> [T_s]
  H_rh/1 -> [H_rh]
  rho_rh/1 -> [rho_rh]
  Unit Delay7/1 -> [P_rh]
  RH Pressure/1 -> Unit Delay7/1
  Unit Delay1/1 -> [W_rh]
  Unit Delay2/1 -> [H_g]
  W_vrh/1 -> [W_vrh]
  Q_rh/1 -> [Q_rh]
  RH H_liq/1 -> Unit Delay2/1
  Unit Delay3/1 -> [T_rh]
  [W_rh] -> Flow to LP Turbine/1
  Mux1/1 -> To Workspace/1
  [W_v] -> Mux1/1
  [W_ms] -> Mux1/2
  [W_rh] -> Mux1/8
  [W_vrh] -> Mux1/10
  [T_s] -> Mux1/3
  [T_rh] -> Mux1/12
  [Q_rh] -> Mux1/11
  [P_rh] -> Mux1/7
  [rho_rh] -> Mux1/5
  [drho_rh_dt] -> Mux1/4
  [H_rh] -> Mux1/6
  [H_g] -> Mux1/9
  [W_vrh] -> Flow to Feedwater Heater 2/1
  [P_rh] -> Steam Pressure Reheater/1
  [H_rh] -> Steam Enthalpy Reheater/1
  [W_ms] -> Minus/1
  [W_rh] -> Minus/2
  Constant/1 -> [V_rh]
  Minus/1 -> Divide/1
  [V_rh] -> Divide/2
  Divide/1 -> rho_rh/1, [drho_rh_dt]
  Divide1/1 -> Minus1/1
  Divide2/1 -> Minus1/2
  [rho_rh] -> Product1/2, Square/1
  Square/1 -> Product/1
  Product1/1 -> Divide1/2
  Product/1 -> Divide2/3
  [V_rh] -> Product1/1
  [V_rh] -> Product/2
  Minus2/1 -> Divide2/2
  [P_rh] -> Divide2/1
  [W_rh] -> Minus2/2
  [W_ms] -> Minus2/1
  [Q_rh] -> Minus3/1
  Product2/1 -> Minus3/2
  Product3/1 -> Minus3/3
  Minus3/1 -> Divide1/1
  [W_ms] -> Product2/1
  [H_g] -> Product2/2
  [W_rh] -> Product3/1
  [H_rh] -> Product3/2
  Minus1/1 -> H_rh/1  "dH_rh/dt"
  [H_rh] -> RH Pressure/1
  [rho_rh] -> RH Pressure/2
  [P_rh] -> Product4/1
  [rho_rh] -> Product4/2
  Product4/1 -> Sqrt/1
  Sqrt/1 -> Product5/2
  [C_rh_X_A_rh] -> Product5/1
  Product5/1 -> Unit Delay1/1
  [P_rh] -> RH H_liq/1
  Constant2/1 -> [tau_rht]
  [W_v] -> Minus4/1
  [W_vrh] -> Minus4/2
  Minus4/1 -> Divide3/1
  [tau_rht] -> Divide3/2
  Divide3/1 -> W_vrh/1  "dWrvh/dt"
  [W_v] -> Minus5/1
  [W_vrh] -> Minus5/2
  Minus5/1 -> Divide4/1
  Constant3/1 -> [Cp_rh]
  Constant4/1 -> Divide4/5
  [tau_rhs] -> Divide4/4
  [Cp_rh] -> Divide4/3
  Minus6/1 -> Divide4/2
  [T_s] -> Minus6/1
  [T_rh] -> Minus6/2
  [Q_rh] -> Divide5/1
  [tau_rhs] -> Divide5/2
  Divide5/1 -> Minus7/2
  Divide4/1 -> Minus7/1
  Minus7/1 -> Q_rh/1  "dQ_rh/dt"
  Constant5/1 -> [tau_rhs]
  Constant6/1 -> [M_stm]
  Constant7/1 -> [R]
  [P_rh] -> Divide6/1
  Constant8/1 -> Divide6/2
  Product6/1 -> Divide7/2
  [M_stm] -> Divide6/3
  Divide6/1 -> Divide7/1
  Divide7/1 -> Unit Delay3/1
  [R] -> Product6/2
  [rho_rh] -> Product6/1
  Constant1/1 -> [C_rh_X_A_rh]

== system MSBR_Plant/Balance of Plant (BOP)/Secondary Steam Valve ==
  Steam from OTSG : Inport
  Constant : Constant
  Minus : Sum  Inputs=+-
  Product : Product
  Steam Valve Coefficient : Constant  Value=C_v
  Steam to Reheater : Outport  VectorParamsAs1DForOutWhenUnconnected=off
  wires:
  Steam from OTSG/1 -> Product/2
  Product/1 -> Steam to Reheater/1
  Steam Valve Coefficient/1 -> Minus/2
  Constant/1 -> Minus/1
  Minus/1 -> Product/1

== system MSBR_Plant/Nuclear Steam Supply System (NSSS)/Coolant Salt Pumps ==
  Constant : Constant  Value=therm_conv_cool
  Constant2 : Constant  Value=tau_p_c
  Constant4 : Constant  Value=trip_time_c
  Coolant Pump 1 : Subsystem
  Coolant Pump 2 : Subsystem
  Coolant Pump 3 : Subsystem
  Coolant Pump 4 : Subsystem
  Demux : Demux
  Demux2 : Demux
  Demux4 : Demux
  Mux : Mux  Inputs=8
  Out Bus Element : Outport  PortName=Coolant Pumps  Element=Flow and hA Frac
  wires:
  Demux4/4 -> Coolant Pump 4/3(Pump Trip Time)
  Demux4/3 -> Coolant Pump 3/3(Pump Trip Time)
  Demux4/2 -> Coolant Pump 2/3(Pump Trip Time)
  Demux4/1 -> Coolant Pump 1/3(Pump Trip Time)
  Demux/4 -> Coolant Pump 4/2(Thermal Conv)
  Demux/3 -> Coolant Pump 3/2(Thermal Conv)
  Demux/2 -> Coolant Pump 2/2(Thermal Conv)
  Demux2/4 -> Coolant Pump 4/1(Pump Decay Rate)
  Demux2/3 -> Coolant Pump 3/1(Pump Decay Rate)
  Demux2/2 -> Coolant Pump 2/1(Pump Decay Rate)
  Demux/1 -> Coolant Pump 1/2(Thermal Conv)
  Demux2/1 -> Coolant Pump 1/1(Pump Decay Rate)
  Constant4/1 -> Demux4/1
  Constant2/1 -> Demux2/1
  Constant/1 -> Demux/1
  Coolant Pump 4/2(Coolant Heat Transfer Fraction) -> Mux/8
  Coolant Pump 4/1(Coolant Flow Fraction) -> Mux/7
  Coolant Pump 2/2(Coolant Heat Transfer Fraction) -> Mux/4
  Coolant Pump 2/1(Coolant Flow Fraction) -> Mux/3
  Coolant Pump 1/2(Coolant Heat Transfer Fraction) -> Mux/2
  Mux/1 -> Out Bus Element/1
  Coolant Pump 3/2(Coolant Heat Transfer Fraction) -> Mux/6
  Coolant Pump 3/1(Coolant Flow Fraction) -> Mux/5
  Coolant Pump 1/1(Coolant Flow Fraction) -> Mux/1
